simulink model "Odd_Slope_Nonlinearity_test"  (Simulink 7.3)
settings: Solver=ode45  StartTime=0.0  StopTime=10.0  RelTol=1e-3
settings Model: Creator=MD710  LastModifiedBy=MD710
settings DebuggingCC: SaveWithParameterizedLinksMsg=none  SolverPrmCheckMsg=none  MultiTaskDSMMsg=warning  MultiTaskCondExecSysMsg=none  FcnCallInpInsideContextMsg=Enable All  StrictBusMsg=None
settings HardwareCC: TargetHWDeviceType=32-bit Generic
settings RTWCC: IncludeERTFirstTime=on
settings GRTTargetCC: TargetFcnLib=ansi_tfl_tmw.mat

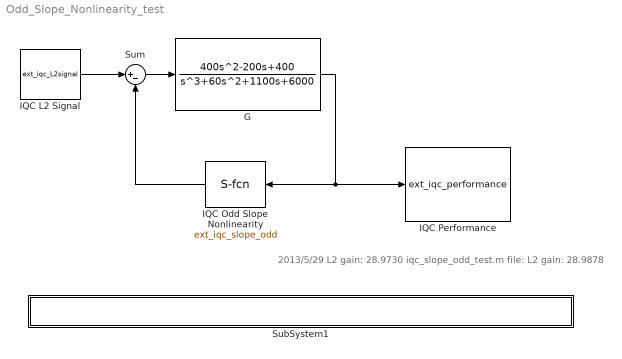
== system Odd_Slope_Nonlinearity_test ==
  note: 2013/5/29 L2 gain: 28.9730
      | iqc_slope_odd_test.m file: L2 gain: 28.9878
  G : TransferFcn  Numerator=[400 -200 400]  Denominator=[1 60 1100 6000]
  IQC L2 Signal : M-S-Function  FunctionName=ext_iqc_L2signal  Parameters=sig_size,sam_time,sig_type,tru_time,sig_amp,sig_fre,user_cus  mask(IQC L2 signal(ver:0.1)){sig_size=1, sam_time=0, sig_type=Step, tru_time=10, sig_amp=1, sig_fre=1, user_cus='2*exp(3*t)'}
      mask prompts: sig_size "Signal Dimension:(Default: 1)"; sam_time "Sample Time:(Default: 0)"; sig_type "Signal Type:"; tru_time "Truncation Time:"; sig_amp "Maximum Amplitude:"; sig_fre "Frequency:"; user_cus "Custom:"
      mask help:
      | Important:
      | In IQC procedure step (as commond iqc_gain_tbx, the task is get
      | L2 gain value), regardless of the user to choose which option (ex sine...),
      | here regarded as generalized L2 signal.
      mask StyleString: edit,edit,popup(Step|Square wave|Sine wave|Custom|Random|External),edit,edit,edit,edit
      mask CallbackString: ||iqc_block_cho(gcb,'L2signal_type')||||
      mask TabNameString: Generalized Parameters,Generalized Parameters,Simulink Parameters,Simulink Parameters,Simulink Parameters,Simulink Parameters,Simulink Parameters
      mask Display: plot(0:0.1:10,[sin(0:0.1:6.2) zeros(1,38)])
  IQC Odd Slope Nonlinearity : M-S-Function  FunctionName=ext_iqc_slope_odd  Parameters=pole,len_def_h,low_bou,upp_bou,out_var  mask(IQC Odd Slope Nonlinearity(ver:0.1)){pole=[-1], len_def_h=1, low_bou=0, upp_bou=1, out_var=''}
      mask prompts: pole "Pole:(Default: [1])"; len_def_h "Length of The Expansion that Defines H:(Default: 0)"; low_bou "Lower Bound on Slope:(Default: 0)"; upp_bou "Upper Bound on Slope:(Default: 1)"; out_var "Output Variable:(Default: empty)"
      mask help:
      | Example: [w,h0,H,xp,xm]=iqc_slope_odd(v,a,N,alpha,beta)
      | Pole:
      |          [a]
      | Length of The Expansion that Defines H:
      |           N
      | Lower Bound on Slope:
      |         alpha
      | Upper Bound on Slope:
      |         beta
      | Output Variable:
      |    {'h0','H','xp','xm'}
      mask Help: eval('doc iqc_slope_odd')
      mask Display: plot(0,0,100,100,[96,2],[50,50],[50,50],[95,4],[97,80,60,40,20,4],[90,90,71,30,10,10],[81,84,60,75,60],[72,71,71,99,71],[81,84],[69,71],[73,75],[97,99],[75,75,75],[96,99,99]);
  IQC Performance : M-S-Function  FunctionName=ext_iqc_performance  Parameters=imp_met,save_lin_com,isiqcbode,fre_ran,uselmitool,lmi_par  mask(IQC Performance(ver:0.1)){imp_met=Only Calculation, save_lin_com=off, isiqcbode=off, fre_ran='', uselmitool=lmilab, lmi_par=''}
      mask prompts: imp_met "Implementation Methods"; save_lin_com "Save the Linear File and Command File"; isiqcbode "Display IQC Bode Figure"; fre_ran "Frequency Range:(Default: empty)"; uselmitool "LMI Tool:"; lmi_par "Parameter:(if empty use define)"
      mask help:
      | Important:
      | In IQC toolbox calculate step (as commond iqc_gain_tbx, the task is get
      | L2 gain value), regardless of the user to connect any signal input(Even if
      | not a signal), here regarded as generalized L2 signal.
      |
      | Example 1: setlmioptions('',[0 200 0 0 777])
      | the block parameter is
      | LMI Tool: lmilab
      | Parameter:
      |        [0 200 0 0 777]
      |
      | Example 2: setlmioptions('yalmip','solver','sdpt3','verbose',1)
      | the block parameter is
      | LMI Tool: yalmip
      | Parameter:
      |        {'solver',sdpt3','verbose',1}
      mask Help:
      | <a href="matlab:doc abst_init_iqc;">abst_init_iqc</a>
      | <a href="matlab:doc setlmioptions;">setlmioptions</a>
      | <a href="matlab:doc iqc_gain_tbx;">iqc_gain_tbx</a>
      mask StyleString: popup(Calculation and Simulation|Only Calculation|Only Simulation),checkbox,checkbox,edit,popup(lmilab|yalmip),edit
      mask CallbackString: iqc_block_cho(gcb,'performance_imp')||iqc_block_cho(gcb,'performance_bodefre')|||
      mask TabNameString: Parameter,Parameter,Parameter,Parameter,LMI Parameter,LMI Parameter
      mask Display: fprintf('In -> Out \n performance \n L2 gain:\n%4.4f',28.973);
  SubSystem1 : Subsystem  mask{filename=iqc_slope_odd_test.m}
      mask init:
      | x_dir=which(filename);
      | x=x_dir;
      settings: OpenFcn=|
      | x_dir=which('iqc_slope_odd_test.m');
      | x=x_dir;
      | edit(x);
      mask Display: disp(['MATLAB file: ' x]);
  Sum : Sum  Inputs=|+-
  wires:
  IQC L2 Signal/1 -> Sum/1
  Sum/1 -> G/1
  IQC Odd Slope Nonlinearity/1 -> Sum/2
  G/1 -> IQC Performance/1, IQC Odd Slope Nonlinearity/1

== system Odd_Slope_Nonlinearity_test/SubSystem1 ==
